simulink model "MotorSim"  (R2021b)
settings: Solver=FixedStepAuto  StartTime=0.0  StopTime=20  FixedStep=0.1  RelTol=1e-3
settings Model: Creator=Ian Lee  LastModifiedBy=Ian Lee

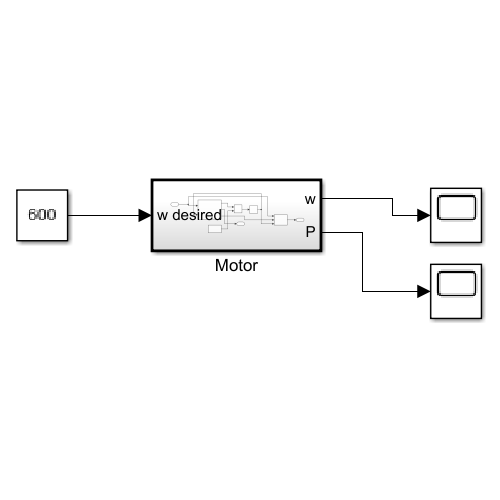
[thumbnail: Simulink's stored preview of the top-level diagram]
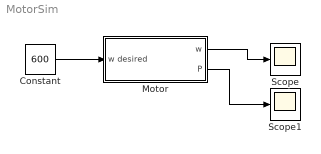
== system MotorSim ==
  Constant : Constant  Value=600
  Motor : Subsystem  TreatAsAtomicUnit=on
  Scope : Scope
  Scope1 : Scope
  wires:
  Motor/1(w) -> Scope/1
  Motor/2(P) -> Scope1/1
  Constant/1 -> Motor/1(w desired)

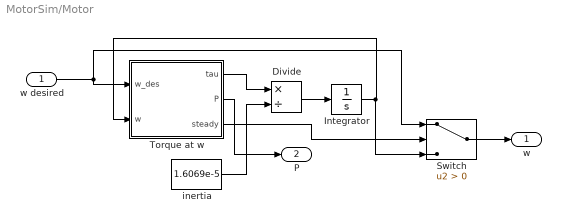
== system MotorSim/Motor ==
  w desired : Inport
  Divide : Product  Inputs=*/
  Integrator : Integrator
  Switch : Switch  Criteria=u2 > Threshold
  Torque at w : MATLAB Function  TreatAsAtomicUnit=on
  inertia : Constant  Value=1.6069e-5
  w : Outport
  P : Outport  Port=2
  wires:
  Torque at w/1(tau) -> Divide/1
  inertia/1 -> Divide/2
  Divide/1 -> Integrator/1
  Integrator/1 -> Switch/3, Torque at w/2(w)
  w desired/1 -> Switch/1, Torque at w/1(w_des)
  Torque at w/2(P) -> P/1
  Torque at w/3(steady) -> Switch/2
  Switch/1 -> w/1

== matlab function MotorSim/Motor/Torque at w ==
  data: w_des input; w input; tau output; P output; steady output
function [tau,P,steady] = fcn(w_des, w)

n = 16577; % slope of w-torque curve (min^-1/mNm)
T_0 = 0.953; % stall torque (mNm)
C_v = 3.42e-6; % dynamic friction torque (mNm/min^-1)
I_0 = 0.019; % No-load current (A)
k_I = 0.281; % current constant (A/mNm)
V = 6; % V
deadzone = 2; % (rad/s)
rpm = abs((w * 60) / (2 * pi));

if(abs(w - w_des) < deadzone)
    tau = 0;
    I = I_0 + k_I * (C_v * rpm);
    P = I * V;
    steady = 1;
else
    T = -((rpm - n * T_0) / n) - C_v * rpm;
    if(w < w_des)
        tau = T / 1000;
    else
        tau = -T / 1000;
    end
    I = I_0 + k_I * T;
    P = I * V;
    steady = 0;
end
